simulink model "PubIfDecisionTOS_MDL"  (R2020b)
settings: configuration reference "DspaceConfig" (kept outside this file)
PostLoadFcn:
  | if any(exist('dsrtsu_mdlpostloadfcn', 'file') ~= 0), dsrtsu_mdlpostloadfcn('Execute', bdroot); end
InitFcn:
  | , if any(exist('dsmpb_private', 'file') ~= 0), dsmpb_private('dsmpb_mdlclblib', 'Init', bdroot); end,
undefined symbols (not defined in the file or in its folder): C_TOS_ACCEgoRAxletoFbumplength_m, C_TOS_ACCTargetFront_Flag, C_TOS_AEBJAPedObjDxThre_Val, C_TOS_AEBJAPedObjDyThre_Val, C_TOS_AEBJATargetSize_Val, C_TOS_AEBJAVehObjDxThre_Val, C_TOS_AEBJAVehObjDyThre_Val, C_TOS_AEBJuncPedTargetSize_Val, C_TOS_AEBLatObjDxThre_Val, C_TOS_AEBLatPedDyThre_Val, C_TOS_AEBLatTargetSize_Val, C_TOS_AEBLongTargetInEgoFront_Flag, C_TOS_axAbsGround_Parameter, C_TOS_CameraConfirmedFlag, C_TOS_CNsubjWidth, C_TOS_CurrentLaneCoreMinWidth_Val, C_TOS_CutInProb_Val_Zero, C_TOS_CutOutProb_Val_Zero, C_TOS_D2R_Val, C_TOS_DefaultValueObjectToCenterLine_dy, C_TOS_EgoCarWidth_Val, C_TOS_EgoDxRefPoint_m, C_TOS_EgoRAxletoFbumplength_m, C_TOS_HalfWidthVehicle_Con, C_TOS_HWA_CurrentLaneFlag, C_TOS_HWA_LeftLaneFlag, C_TOS_HWA_MovingDir_Vaild, C_TOS_HWA_MovState_Vaild, C_TOS_HWA_RightLaneFlag, C_TOS_LaneLineCourseErrorFront, C_TOS_LaneLineCourseErrorRear, C_TOS_MotorbikeDefaultWidth_m, C_TOS_NumberOfEffectiveTargets, C_TOS_Obj_Age_Val, C_TOS_Objdx_Constraint_Val, C_TOS_ObjectDefaultWidth_m, C_TOS_ObjInCurrentLane_Val, C_TOS_ObjInCurrentLaneValid, C_TOS_ObjInLeftLaneValid, C_TOS_ObjInRightLaneValid, C_TOS_ObjNotInCurrentLane_Val, C_TOS_ObjNotREElementType, C_TOS_ObjPredictDis_dy_ConstantVal_Zeros, C_TOS_ObjToCenterLine_ConstantVal_Zeros, C_TOS_OFMObjIDInvilad_Val, C_TOS_PIL_LatDisCons_Val_zero, C_TOS_PIL_ObjectCutInFlag_b, C_TOS_PIL_ObjectCutOutFlag_b, C_TOS_PIL_ObjLaneProb_al_Val, C_TOS_PP_ObjFusType_FC_Confirm_b, C_TOS_PP_ObjFusType_FC_FR_Confirm_b, C_TOS_PP_ObjFusType_FR_Confirm_b, C_TOS_RE_80BoolDefault_Val, C_TOS_RE_80Single181Default_Val, C_TOS_RE_80Single255Default_Val, C_TOS_RE_80Uint8Default_Val, C_TOS_RE_D2R, C_TOS_RE_D_180_Val, C_TOS_RE_InvalidObjectID_Val, C_TOS_RE_InvalidTargetChainDir_Val ... (+142)
libraries: simulink x1650, TOS_LIB x361, canfdmsglib x14
(part 49 of 69)

== system PubIfDecisionTOS_MDL/TOS_20201112/TOS_2012080320/TOS/LC_LCKie_ELK/TOS_HWA/CurrentLane/HWA_Object_PreConfirm/TOS_HWA_CurrentLaneFront_TargPreConfirm/TOS_HWA_CurrentLaneFront_TargPreConfirm/Subsystem3 ==
  FR_Confirm : Inport
  Obj_MovingState : Inport  Port=2
  Object_ObstacleProb : Inport  Port=3
  Object_DY : Inport  Port=4
  Chart : Stateflow chart  TreatAsAtomicUnit=on
  Data Type Conversion1 : DataTypeConversion  OutDataTypeStr=Enum: OFM_OBJ_MOVINGSTATE_E
  TOS_HWA_TargetPre_FenceFlag : Outport
  wires:
  Chart/1(ObjectisFence_Flag) -> TOS_HWA_TargetPre_FenceFlag/1
  Object_DY/1 -> Chart/4(Object_DY)
  FR_Confirm/1 -> Chart/1(FR_Confirm)
  Obj_MovingState/1 -> Data Type Conversion1/1
  Object_ObstacleProb/1 -> Chart/3(Object_ObstacleProb)
  Data Type Conversion1/1 -> Chart/2(Obj_MovingState)

== system PubIfDecisionTOS_MDL/TOS_20201112/TOS_2012080320/TOS/LC_LCKie_ELK/TOS_HWA/CurrentLane/HWA_Object_PreConfirm/TOS_HWA_CurrentLaneFront_TargPreConfirm/TOS_HWA_CurrentLaneFront_TargPreConfirm/TOS_HWA_DyConfirm ==
  TOS_HWA_Dy : Inport
  Abs : Abs
  Abs1 : Abs
  Bus Selector3 : BusSelector  OutputSignals=PIL_OverlapRatio,Object_DY,Obj_Dx,Object_ObjType
  Compare To Constant1 : simulink/Logic and Bit Operations/Compare To Constant  relop===  const=OFM_OBJ_TYPE_E.UNKNOWN_TYPE  OutDataTypeStr=boolean
      settings: AttributesFormatString=OFM_OBJ_TYPE_E.UNKNOWN_TYPE = 1
  Compare To Constant2 : simulink/Logic and Bit Operations/Compare To Constant  relop===  const=OFM_OBJ_TYPE_E.MOTORBIKE  OutDataTypeStr=boolean
      settings: AttributesFormatString=OFM_OBJ_TYPE_E.MOTORBIKE = 4
  Compare To Constant3 : simulink/Logic and Bit Operations/Compare To Constant  relop===  const=OFM_OBJ_TYPE_E.PEDESTRIAN  OutDataTypeStr=boolean
      settings: AttributesFormatString=OFM_OBJ_TYPE_E.PEDESTRIAN = 6
  Compare To Constant4 : simulink/Logic and Bit Operations/Compare To Constant  relop===  const=OFM_OBJ_TYPE_E.BICYCLE  OutDataTypeStr=boolean
      settings: AttributesFormatString=OFM_OBJ_TYPE_E.BICYCLE = 5
  Compare To Constant5 : simulink/Logic and Bit Operations/Compare To Constant  relop===  const=OFM_OBJ_TYPE_E.GENERAL_OBJECT  OutDataTypeStr=boolean
      settings: AttributesFormatString=OFM_OBJ_TYPE_E.GENERAL_OBJECT = 7
  Compare To Constant6 : simulink/Logic and Bit Operations/Compare To Constant  relop===  const=OFM_OBJ_TYPE_E.ANIMAL  OutDataTypeStr=boolean
      settings: AttributesFormatString=OFM_OBJ_TYPE_E.ANIMAL = 8
  Compare To Constant7 : simulink/Logic and Bit Operations/Compare To Constant  relop=>=  const=P_TOS_HWA_TargetPre_OverlapThre_Val  OutDataTypeStr=boolean
      settings: AttributesFormatString=P_TOS_HWA_TargetPre_OverlapThre_Val = 0.05
  Data Type Conversion2 : DataTypeConversion  OutDataTypeStr=Enum: OFM_OBJ_TYPE_E
  Logical Operator1 : Logic  Operator=OR  Inputs=6  AllPortsSameDT=off  OutDataTypeStr=boolean
  Logical Operator2 : Logic  Operator=NOT  Inputs=1  AllPortsSameDT=off  OutDataTypeStr=boolean
  Logical Operator3 : Logic  Inputs=3  AllPortsSameDT=off  OutDataTypeStr=boolean
  Logical Operator4 : Logic  AllPortsSameDT=off  OutDataTypeStr=boolean
  Logical Operator6 : Logic  Operator=OR  AllPortsSameDT=off  OutDataTypeStr=boolean
  Relational Operator : RelationalOperator  Operator=<=  OutDataTypeStr=boolean  RndMeth=Simplest
  data3 : Lookup_n-D  NumberOfTableDimensions=1  BreakpointsForDimension1=[0,20,40,60,80,100,120,140]  Table=[1.4,1.4,1.3,1.3,1.2,1.2,1.2,1.2]  RndMeth=Simplest  InputSameDT=on
  TOS_HWA_DyConfirm : Outport
  wires:
  Logical Operator6/1 -> TOS_HWA_DyConfirm/1
  TOS_HWA_Dy/1 -> Bus Selector3/1
  Relational Operator/1 -> Logical Operator3/2
  Abs/1 -> data3/1
  data3/1 -> Relational Operator/2
  Abs1/1 -> Relational Operator/1
  Compare To Constant3/1 -> Logical Operator1/1
  Bus Selector3/2 -> Abs1/1  "<Object_DY>"
  Data Type Conversion2/1 -> Compare To Constant1/1, Compare To Constant2/1, Compare To Constant4/1, Compare To Constant5/1, Compare To Constant6/1, Compare To Constant3/1
  Compare To Constant1/1 -> Logical Operator1/2
  Compare To Constant2/1 -> Logical Operator1/3
  Compare To Constant4/1 -> Logical Operator1/4
  Compare To Constant5/1 -> Logical Operator1/5
  Compare To Constant6/1 -> Logical Operator1/6
  Logical Operator1/1 -> Logical Operator2/1, Logical Operator3/3
  Bus Selector3/3 -> Abs/1  "<Obj_Dx>"
  Bus Selector3/4 -> Data Type Conversion2/1  "<Object_ObjType>"
  Bus Selector3/1 -> Compare To Constant7/1  "<PIL_OverlapRatio>"
  Compare To Constant7/1 -> Logical Operator3/1, Logical Operator4/2
  Logical Operator2/1 -> Logical Operator4/1
  Logical Operator4/1 -> Logical Operator6/1
  Logical Operator3/1 -> Logical Operator6/2

== system PubIfDecisionTOS_MDL/TOS_20201112/TOS_2012080320/TOS/LC_LCKie_ELK/TOS_HWA/LeftLane/HWA_Object_PreConfirm/HWA_Object_PreConfirm/HWA_Object_PreConfirm/  ==
  Object_Type : Inport
  Compare To Constant : simulink/Logic and Bit Operations/Compare To Constant  relop===  const=OFM_OBJ_TYPE_E.CAR  OutDataTypeStr=boolean
      settings: AttributesFormatString=OFM_OBJ_TYPE_E.CAR = 2
  Compare To Constant1 : simulink/Logic and Bit Operations/Compare To Constant  relop===  const=OFM_OBJ_TYPE_E.TRUCK  OutDataTypeStr=boolean
      settings: AttributesFormatString=OFM_OBJ_TYPE_E.TRUCK = 3
  Compare To Constant2 : simulink/Logic and Bit Operations/Compare To Constant  relop===  const=OFM_OBJ_TYPE_E.UNKNOWN_TYPE  OutDataTypeStr=boolean
      settings: AttributesFormatString=OFM_OBJ_TYPE_E.UNKNOWN_TYPE = 1
  Compare To Constant3 : simulink/Logic and Bit Operations/Compare To Constant  relop===  const=OFM_OBJ_TYPE_E.PEDESTRIAN  OutDataTypeStr=boolean
      settings: AttributesFormatString=OFM_OBJ_TYPE_E.PEDESTRIAN = 6
  Compare To Constant4 : simulink/Logic and Bit Operations/Compare To Constant  relop===  const=OFM_OBJ_TYPE_E.MOTORBIKE  OutDataTypeStr=boolean
      settings: AttributesFormatString=OFM_OBJ_TYPE_E.MOTORBIKE = 4
  Compare To Constant5 : simulink/Logic and Bit Operations/Compare To Constant  relop===  const=OFM_OBJ_TYPE_E.BICYCLE  OutDataTypeStr=boolean
      settings: AttributesFormatString=OFM_OBJ_TYPE_E.BICYCLE = 5
  Compare To Constant6 : simulink/Logic and Bit Operations/Compare To Constant  relop===  const=OFM_OBJ_TYPE_E.GENERAL_OBJECT  OutDataTypeStr=boolean
      settings: AttributesFormatString=OFM_OBJ_TYPE_E.GENERAL_OBJECT = 7
  Compare To Constant7 : simulink/Logic and Bit Operations/Compare To Constant  relop===  const=OFM_OBJ_TYPE_E.ANIMAL  OutDataTypeStr=boolean
      settings: AttributesFormatString=OFM_OBJ_TYPE_E.ANIMAL = 8
  Data Type Conversion : DataTypeConversion  OutDataTypeStr=Enum: OFM_OBJ_TYPE_E
  Logical Operator1 : Logic  Operator=OR  Inputs=8  AllPortsSameDT=off  OutDataTypeStr=boolean
  TOS_HWA_TargetPre_ObjType : Outport
  wires:
  Object_Type/1 -> Data Type Conversion/1
  Data Type Conversion/1 -> Compare To Constant6/1, Compare To Constant7/1, Compare To Constant3/1, Compare To Constant5/1, Compare To Constant4/1, Compare To Constant1/1, Compare To Constant/1, Compare To Constant2/1
  Compare To Constant/1 -> Logical Operator1/2
  Compare To Constant1/1 -> Logical Operator1/3
  Compare To Constant4/1 -> Logical Operator1/4
  Compare To Constant5/1 -> Logical Operator1/5
  Logical Operator1/1 -> TOS_HWA_TargetPre_ObjType/1
  Compare To Constant2/1 -> Logical Operator1/1
  Compare To Constant3/1 -> Logical Operator1/6
  Compare To Constant6/1 -> Logical Operator1/7
  Compare To Constant7/1 -> Logical Operator1/8

== system PubIfDecisionTOS_MDL/TOS_20201112/TOS_2012080320/TOS/LC_LCKie_ELK/TOS_HWA/LeftLane/HWA_Object_PreConfirm/HWA_Object_PreConfirm/HWA_Object_PreConfirm/Subsystem ==
  PP_ObjFusType_FC_FR_Confirm : Inport
  PP_ObjFusType_FR_Confirm : Inport  Port=2
  PP_ObjFusType_FC_Confirm : Inport  Port=3
  Compare To Constant1 : simulink/Logic and Bit Operations/Compare To Constant  relop===  const=C_TOS_PP_ObjFusType_FC_Confirm_b  OutDataTypeStr=boolean
      settings: AttributesFormatString=C_TOS_PP_ObjFusType_FC_Confirm_b = 1
  Compare To Constant5 : simulink/Logic and Bit Operations/Compare To Constant  relop===  const=C_TOS_PP_ObjFusType_FC_FR_Confirm_b  OutDataTypeStr=boolean
      settings: AttributesFormatString=C_TOS_PP_ObjFusType_FC_FR_Confirm_b = 1
  Compare To Constant6 : simulink/Logic and Bit Operations/Compare To Constant  relop===  const=C_TOS_PP_ObjFusType_FR_Confirm_b  OutDataTypeStr=boolean
      settings: AttributesFormatString=C_TOS_PP_ObjFusType_FR_Confirm_b = 1
  Logical Operator : Logic  Operator=OR  Inputs=3  AllPortsSameDT=off  OutDataTypeStr=boolean
  TOS_HWA_TargetPre_TargetFusionTypeFlag : Outport
  wires:
  Logical Operator/1 -> TOS_HWA_TargetPre_TargetFusionTypeFlag/1
  Compare To Constant1/1 -> Logical Operator/3
  Compare To Constant6/1 -> Logical Operator/2
  PP_ObjFusType_FC_FR_Confirm/1 -> Compare To Constant5/1
  PP_ObjFusType_FC_Confirm/1 -> Compare To Constant1/1
  PP_ObjFusType_FR_Confirm/1 -> Compare To Constant6/1
  Compare To Constant5/1 -> Logical Operator/1

== system PubIfDecisionTOS_MDL/TOS_20201112/TOS_2012080320/TOS/LC_LCKie_ELK/TOS_HWA/LeftLane/HWA_Object_PreConfirm/HWA_Object_PreConfirm/HWA_Object_PreConfirm/Subsystem1 ==
  note: 静止目标 、必须有摄像头参与
  PP_ObjFusType_FC_Confirm : Inport
  Obj_MovingState : Inport  Port=2
  Compare To Constant2 : simulink/Logic and Bit Operations/Compare To Constant  relop===  const=OFM_OBJ_MOVINGSTATE_E.UNKNOWN  OutDataTypeStr=boolean
      settings: AttributesFormatString=OFM_OBJ_MOVINGSTATE_E.UNKNOWN = 1
  Compare To Constant3 : simulink/Logic and Bit Operations/Compare To Constant  relop===  const=OFM_OBJ_MOVINGSTATE_E.STATIONARY  OutDataTypeStr=boolean
      settings: AttributesFormatString=OFM_OBJ_MOVINGSTATE_E.STATIONARY = 3
  Compare To Constant5 : simulink/Logic and Bit Operations/Compare To Constant  relop===  const=C_TOS_PP_ObjFusType_FC_Confirm_b  OutDataTypeStr=boolean
      settings: AttributesFormatString=C_TOS_PP_ObjFusType_FC_Confirm_b = 1
  Constant : Constant  OutDataTypeStr=boolean
  Data Type Conversion1 : DataTypeConversion  OutDataTypeStr=Enum: OFM_OBJ_MOVINGSTATE_E
  Logical Operator : Logic  AllPortsSameDT=off  OutDataTypeStr=boolean
  Logical Operator4 : Logic  Operator=OR  AllPortsSameDT=off  OutDataTypeStr=boolean
  Switch : Switch  Criteria=u2 > Threshold
  TOS_HWA_TargetPre_ObjectPassedbyTarget_Flag : Outport
  wires:
  Switch/1 -> TOS_HWA_TargetPre_ObjectPassedbyTarget_Flag/1
  Compare To Constant3/1 -> Logical Operator4/1
  Obj_MovingState/1 -> Data Type Conversion1/1
  Data Type Conversion1/1 -> Compare To Constant2/1, Compare To Constant3/1
  PP_ObjFusType_FC_Confirm/1 -> Compare To Constant5/1
  Compare To Constant5/1 -> Logical Operator/1
  Compare To Constant2/1 -> Logical Operator4/2
  Logical Operator4/1 -> Logical Operator/2, Switch/2
  Logical Operator/1 -> Switch/1
  Constant/1 -> Switch/3

== system PubIfDecisionTOS_MDL/TOS_20201112/TOS_2012080320/TOS/LC_LCKie_ELK/TOS_HWA/LeftLane/HWA_Object_PreConfirm/HWA_Object_PreConfirm/HWA_Object_PreConfirm/TOS_HWA_DyConfirm ==
  TOS_HWA_Dy : Inport
  Abs : Abs
  Abs1 : Abs
  Bus Selector3 : BusSelector  OutputSignals=Object_DY,Obj_Dx,Object_ObjType
  Compare To Constant : simulink/Logic and Bit Operations/Compare To Constant  relop===  const=OFM_OBJ_TYPE_E.CAR  OutDataTypeStr=boolean
      settings: AttributesFormatString=OFM_OBJ_TYPE_E.CAR = 2
  Compare To Constant1 : simulink/Logic and Bit Operations/Compare To Constant  relop===  const=OFM_OBJ_TYPE_E.TRUCK  OutDataTypeStr=boolean
      settings: AttributesFormatString=OFM_OBJ_TYPE_E.TRUCK = 3
  Compare To Constant4 : simulink/Logic and Bit Operations/Compare To Constant  relop===  const=OFM_OBJ_TYPE_E.MOTORBIKE  OutDataTypeStr=boolean
      settings: AttributesFormatString=OFM_OBJ_TYPE_E.MOTORBIKE = 4
  Compare To Constant5 : simulink/Logic and Bit Operations/Compare To Constant  relop===  const=OFM_OBJ_TYPE_E.BICYCLE  OutDataTypeStr=boolean
      settings: AttributesFormatString=OFM_OBJ_TYPE_E.BICYCLE = 5
  Data Type Conversion2 : DataTypeConversion  OutDataTypeStr=Enum: OFM_OBJ_TYPE_E
  Logical Operator1 : Logic  Operator=OR  Inputs=4  AllPortsSameDT=off  OutDataTypeStr=boolean
  Logical Operator2 : Logic  Operator=OR  AllPortsSameDT=off  OutDataTypeStr=boolean
  Relational Operator : RelationalOperator  Operator=<=  OutDataTypeStr=boolean  RndMeth=Simplest
  data3 : Lookup_n-D  NumberOfTableDimensions=1  BreakpointsForDimension1=[0,20,40,60,80,100,120,140]  Table=[1.4,1.4,1.3,1.3,1.2,1.2,1.2,1.2]  RndMeth=Simplest  InputSameDT=on
  TOS_HWA_TargetPre_DyConfirm : Outport
  wires:
  Logical Operator2/1 -> TOS_HWA_TargetPre_DyConfirm/1
  TOS_HWA_Dy/1 -> Bus Selector3/1
  Relational Operator/1 -> Logical Operator2/1
  Abs/1 -> data3/1
  data3/1 -> Relational Operator/2
  Abs1/1 -> Relational Operator/1
  Bus Selector3/1 -> Abs1/1  "<Object_DY>"
  Data Type Conversion2/1 -> Compare To Constant/1, Compare To Constant5/1, Compare To Constant4/1, Compare To Constant1/1
  Logical Operator1/1 -> Logical Operator2/2
  Bus Selector3/2 -> Abs/1  "<Obj_Dx>"
  Bus Selector3/3 -> Data Type Conversion2/1  "<Object_ObjType>"
  Compare To Constant/1 -> Logical Operator1/1
  Compare To Constant1/1 -> Logical Operator1/2
  Compare To Constant4/1 -> Logical Operator1/3
  Compare To Constant5/1 -> Logical Operator1/4

== system PubIfDecisionTOS_MDL/TOS_20201112/TOS_2012080320/TOS/LC_LCKie_ELK/TOS_HWA/LeftLane/TOS_HWA_LeftLane/TOS_HWA_LeftLane/TOS_HWA/HWA_LeftLane ==
  Object_VX : Inport
  Object_VY : Inport  Port=2
  object_MovingState : Inport  Port=3
  PP_ObjMovingDirSignalProcessing : Inport  Port=4
  Object_HeadingAngle : Inport  Port=5
  Object_Type : Inport  Port=6
  TOS_TLJ_LeftLaneConfirm_Flag : Inport  Port=7
  Object_DX : Inport  Port=8
  Object_DY : Inport  Port=9
  Object_Fus_Type : Inport  Port=10
  PP_ObjFusType_FC_FR_Confirm : Inport  Port=11
  PP_ObjFusType_FR_Confirm : Inport  Port=12
  PP_ObjFusType_FC_Confirm : Inport  Port=13
  VIE_EgoVelocity : Inport  Port=14
  Bus Creator : BusCreator  Inputs=14
  Bus Creator1 : BusCreator  Inputs=3
  Bus Creator2 : BusCreator  Inputs=10
  Bus Creator3 : BusCreator  Inputs=10
  Bus Creator4 : BusCreator  Inputs=10
  Bus Selector : BusSelector  OutputSignals=object_MovingState,PP_ObjMovingDirSignalProcessing,Object_HeadingAngle,Object_VX,Object_VY,VIE_EgoVelocity
  Bus Selector1 : BusSelector  OutputSignals=Object_VX,Object_VY,VIE_EgoVelocity
  Bus Selector2 : BusSelector  OutputSignals=HWA_MovState_InternalSig,HWA_InternalSig.Object_Fus_Type,HWA_InternalSig.TOS_TLJ_LeftLaneConfirm_Flag,HWA_MovingDir_InternalSig,HWA_InternalSig.Object_DY,HWA_InternalSig.Object_DX
  Bus Selector3 : BusSelector  OutputSignals=HWA_InternalSig.object_MovingState,HWA_InternalSig.PP_ObjFusType_FR_Confirm,HWA_InternalSig.PP_ObjFusType_FC_Confirm,HWA_MovState_InternalSig,HWA_InternalSig.TOS_TLJ_LeftLaneConfirm_Flag,HWA_MovingDir_InternalSig,HWA_InternalSig.Object_DX
  Bus Selector4 : BusSelector  OutputSignals=HWA_InternalSig.Object_DX
  Bus Selector5 : BusSelector  OutputSignals=HWA_InternalSig.Object_DX
  Bus Selector6 : BusSelector  OutputSignals=TOS_HWA_LeftFront_TargConfirm_b,TOS_HWA_LeftRear_TargConfirm_b,TOS_HWA_LeftFront_FusType_ObserVale,TOS_HWA_InLeftLane_Front_Flag_ObserVale,TOS_HWA_LeftFront_TargMovDir_ObserVale,TOS_HWA_LeftRear_MovState_ObserVale,TOS_HWA_LeftRear_FusionType_ObserVale,TOS_HWA_InLeftLane_Rear_Flag_ObserVale,TOS_HWA_LeftRear_TargetMovingDir_ObserVale,TOS_HWA_LeftRear_DyConfirm_ObserVale
  Compare To Constant1 : simulink/Logic and Bit Operations/Compare To Constant  relop=<=  const=P_TOS_EgoFrontDxThre_Val  OutDataTypeStr=boolean
      settings: AttributesFormatString=P_TOS_EgoFrontDxThre_Val = 120
  Compare To Constant14 : simulink/Logic and Bit Operations/Compare To Constant  relop=<  const=P_TOS_RefPoint_dx_m  OutDataTypeStr=boolean
      settings: AttributesFormatString=P_TOS_RefPoint_dx_m = 0
  Compare To Constant2 : simulink/Logic and Bit Operations/Compare To Constant  relop=>=  const=P_TOS_RefPoint_dx_m  OutDataTypeStr=boolean
      settings: AttributesFormatString=P_TOS_RefPoint_dx_m = 0
  Compare To Constant3 : simulink/Logic and Bit Operations/Compare To Constant  relop=>=  const=P_TOS_EgoRearDxThre_Val  OutDataTypeStr=boolean
      settings: AttributesFormatString=P_TOS_EgoRearDxThre_Val = -80
  HWA_LeftLane_Default : Subsystem
  HWA_LeftLane_Front : Subsystem
  HWA_LeftLane_Rear : Subsystem
  HWA_MovState : Subsystem
  HWA_MovingDir : Subsystem
  Logical Operator1 : Logic  AllPortsSameDT=off  OutDataTypeStr=boolean
  Logical Operator2 : Logic  AllPortsSameDT=off  OutDataTypeStr=boolean
  Logical Operator3 : Logic  Operator=OR  AllPortsSameDT=off  OutDataTypeStr=boolean
  Switch : Switch  Criteria=u2 > Threshold
  Switch1 : Switch  Criteria=u2 > Threshold
  TOS_HWA_TargetInLeftLane_b : Outport
  TOS_HWA_LeftFront_TargConfirm_b : Outport  Port=2
  TOS_HWA_LeftRear_TargConfirm_b : Outport  Port=3
  TOS_HWA_LeftFront_FusType_ObserVale : Outport  Port=4
  TOS_HWA_InLeftLane_Front_Flag_ObserVale : Outport  Port=5
  TOS_HWA_LeftFront_TargMovDir_ObserVale : Outport  Port=6
  TOS_HWA_LeftRear_MovState_ObserVale : Outport  Port=7
  TOS_HWA_LeftRear_FusionType_ObserVale : Outport  Port=8
  TOS_HWA_InLeftLane_Rear_Flag_ObserVale : Outport  Port=9
  TOS_HWA_LeftRear_TargetMovingDir_ObserVale : Outport  Port=10
  TOS_HWA_LeftRear_DyConfirm_ObserVale : Outport  Port=11
  wires:
  Bus Selector3/7 -> HWA_LeftLane_Front/7(Object_DX)  "<Object_DX>"
  Logical Operator3/1 -> TOS_HWA_TargetInLeftLane_b/1
  Bus Selector6/10 -> TOS_HWA_LeftRear_DyConfirm_ObserVale/1  "<TOS_HWA_LeftRear_DyConfirm_ObserVale>"
  Bus Selector6/9 -> TOS_HWA_LeftRear_TargetMovingDir_ObserVale/1  "<TOS_HWA_LeftRear_TargetMovingDir_ObserVale>"
  Bus Selector6/8 -> TOS_HWA_InLeftLane_Rear_Flag_ObserVale/1  "<TOS_HWA_InLeftLane_Rear_Flag_ObserVale>"
  Bus Selector6/7 -> TOS_HWA_LeftRear_FusionType_ObserVale/1  "<TOS_HWA_LeftRear_FusionType_ObserVale>"
  Bus Selector6/6 -> TOS_HWA_LeftRear_MovState_ObserVale/1  "<TOS_HWA_LeftRear_MovState_ObserVale>"
  Bus Selector6/5 -> TOS_HWA_LeftFront_TargMovDir_ObserVale/1  "<TOS_HWA_LeftFront_TargMovDir_ObserVale>"
  Bus Selector6/4 -> TOS_HWA_InLeftLane_Front_Flag_ObserVale/1  "<TOS_HWA_InLeftLane_Front_Flag_ObserVale>"
  Bus Selector6/3 -> TOS_HWA_LeftFront_FusType_ObserVale/1  "<TOS_HWA_LeftFront_FusType_ObserVale>"
  Bus Selector6/2 -> TOS_HWA_LeftRear_TargConfirm_b/1, Logical Operator3/2  "<TOS_HWA_LeftRear_TargConfirm_b>"
  Bus Selector6/1 -> TOS_HWA_LeftFront_TargConfirm_b/1, Logical Operator3/1  "<TOS_HWA_LeftFront_TargConfirm_b>"
  Switch/1 -> Bus Selector6/1
  Bus Creator4/1 -> Switch1/3
  Switch1/1 -> Switch/3
  Bus Creator3/1 -> Switch1/1
  Bus Creator2/1 -> Switch/1
  Bus Selector4/1 -> Compare To Constant3/1, Compare To Constant14/1  "<Object_DX>"
  Bus Selector2/6 -> HWA_LeftLane_Rear/6(Object_DX)  "<Object_DX>"
  Bus Selector3/6 -> HWA_LeftLane_Front/6(HWA_MovingDir_InternalSig)  "<HWA_MovingDir_InternalSig>"
  Bus Selector3/5 -> HWA_LeftLane_Front/5(TOS_TLJ_LeftLaneConfirm_Flag)  "<TOS_TLJ_LeftLaneConfirm_Flag>"
  Bus Selector3/4 -> HWA_LeftLane_Front/4(HWA_MovState_InternalSig)  "<HWA_MovState_InternalSig>"
  Bus Selector3/3 -> HWA_LeftLane_Front/3(PP_ObjFusType_FC_Confirm)  "<PP_ObjFusType_FC_Confirm>"
  Bus Selector3/2 -> HWA_LeftLane_Front/2(PP_ObjFusType_FR_Confirm)  "<PP_ObjFusType_FR_Confirm>"
  Bus Selector3/1 -> HWA_LeftLane_Front/1(object_MovingState)  "<object_MovingState>"
  Bus Selector2/1 -> HWA_LeftLane_Rear/1(HWA_MovState_InternalSig)  "<HWA_MovState_InternalSig>"
  Bus Selector2/2 -> HWA_LeftLane_Rear/2(Object_Fus_Type)  "<Object_Fus_Type>"
  Bus Selector2/3 -> HWA_LeftLane_Rear/3(TOS_TLJ_LeftLaneConfirm_Flag)  "<TOS_TLJ_LeftLaneConfirm_Flag>"
  Bus Selector2/4 -> HWA_LeftLane_Rear/4(HWA_MovingDir_InternalSig)  "<HWA_MovingDir_InternalSig>"
  Bus Selector2/5 -> HWA_LeftLane_Rear/5(Object_DY)  "<Object_DY>"
  Object_DY/1 -> Bus Creator/9  "Object_DY"
  Bus Creator1/1 -> Bus Selector3/1, Bus Selector5/1, Bus Selector2/1, Bus Selector4/1
  HWA_MovingDir/1(HWA_MovingDir_InternalSig) -> Bus Creator1/2  "HWA_MovingDir_InternalSig"
  HWA_MovState/1(HWA_MovState_InternalSig) -> Bus Creator1/3  "HWA_MovState_InternalSig"
  Bus Selector1/3 -> HWA_MovState/3(VIE_EgoVelocity)  "<VIE_EgoVelocity>"
  Bus Selector1/2 -> HWA_MovState/2(Object_VY)  "<Object_VY>"
  Bus Selector1/1 -> HWA_MovState/1(Object_VX)  "<Object_VX>"
  Bus Selector/6 -> HWA_MovingDir/6(VIE_EgoVelocity)  "<VIE_EgoVelocity>"
  Bus Selector/5 -> HWA_MovingDir/5(Object_VY)  "<Object_VY>"
  Bus Selector/4 -> HWA_MovingDir/4(Object_VX)  "<Object_VX>"
  Bus Selector/3 -> HWA_MovingDir/3(Object_HeadingAngle)  "<Object_HeadingAngle>"
  Bus Selector/2 -> HWA_MovingDir/2(PP_ObjMovingDirSignalProcessing)  "<PP_ObjMovingDirSignalProcessing>"
  Bus Selector/1 -> HWA_MovingDir/1(object_MovingState)  "<object_MovingState>"
  Bus Creator/1 -> Bus Creator1/1, Bus Selector/1, Bus Selector1/1  "HWA_InternalSig"
  PP_ObjFusType_FR_Confirm/1 -> Bus Creator/12  "PP_ObjFusType_FR_Confirm"
  PP_ObjFusType_FC_FR_Confirm/1 -> Bus Creator/11  "PP_ObjFusType_FC_FR_Confirm"
  Object_Fus_Type/1 -> Bus Creator/10  "Object_Fus_Type"
  Object_DX/1 -> Bus Creator/8  "Object_DX"
  TOS_TLJ_LeftLaneConfirm_Flag/1 -> Bus Creator/7  "TOS_TLJ_LeftLaneConfirm_Flag"
  Object_Type/1 -> Bus Creator/6  "Object_Type"
  Object_HeadingAngle/1 -> Bus Creator/5  "Object_HeadingAngle"
  PP_ObjMovingDirSignalProcessing/1 -> Bus Creator/4  "PP_ObjMovingDirSignalProcessing"
  object_MovingState/1 -> Bus Creator/3  "object_MovingState"
  Object_VY/1 -> Bus Creator/2  "Object_VY"
  VIE_EgoVelocity/1 -> Bus Creator/14  "VIE_EgoVelocity"
  Object_VX/1 -> Bus Creator/1  "Object_VX"
  Logical Operator2/1 -> Switch/2
  Logical Operator1/1 -> Switch1/2
  Compare To Constant1/1 -> Logical Operator2/2
  Compare To Constant2/1 -> Logical Operator2/1
  Compare To Constant14/1 -> Logical Operator1/2
  Compare To Constant3/1 -> Logical Operator1/1
  Bus Selector5/1 -> Compare To Constant2/1, Compare To Constant1/1  "<Object_DX>"
  PP_ObjFusType_FC_Confirm/1 -> Bus Creator/13  "PP_ObjFusType_FC_Confirm"
  HWA_LeftLane_Front/1(TOS_HWA_LeftFront_TargConfirm_b) -> Bus Creator2/1
  HWA_LeftLane_Front/2(TOS_HWA_LeftFront_FusType_ObserVale) -> Bus Creator2/2
  HWA_LeftLane_Front/3(TOS_HWA_InLeftLane_Front_Flag_ObserVale) -> Bus Creator2/3
  HWA_LeftLane_Front/4(TOS_HWA_LeftFront_TargMovDir_ObserVale) -> Bus Creator2/4
  HWA_LeftLane_Front/5(TOS_HWA_LeftRear_TargConfirm_b) -> Bus Creator2/5
  HWA_LeftLane_Front/6(TOS_HWA_LeftRear_MovState_ObserVale) -> Bus Creator2/6
  HWA_LeftLane_Front/7(TOS_HWA_LeftRear_FusionType_ObserVale) -> Bus Creator2/7
  HWA_LeftLane_Front/8(TOS_HWA_InLeftLane_Rear_Flag_ObserVale) -> Bus Creator2/8
  HWA_LeftLane_Front/9(TOS_HWA_LeftRear_TargetMovingDir_ObserVale) -> Bus Creator2/9
  HWA_LeftLane_Front/10(TOS_HWA_LeftRear_DyConfirm_ObserVale) -> Bus Creator2/10
  HWA_LeftLane_Rear/1(TOS_HWA_LeftFront_TargConfirm_b) -> Bus Creator3/1
  HWA_LeftLane_Rear/2(TOS_HWA_LeftFront_FusType_ObserVale) -> Bus Creator3/2
  HWA_LeftLane_Rear/3(TOS_HWA_InLeftLane_Front_Flag_ObserVale) -> Bus Creator3/3
  HWA_LeftLane_Rear/4(TOS_HWA_LeftFront_TargMovDir_ObserVale) -> Bus Creator3/4
  HWA_LeftLane_Rear/5(TOS_HWA_LeftRear_TargConfirm_b) -> Bus Creator3/5
  HWA_LeftLane_Rear/6(TOS_HWA_LeftRear_MovState_ObserVale) -> Bus Creator3/6
  HWA_LeftLane_Rear/7(TOS_HWA_LeftRear_FusionType_ObserVale) -> Bus Creator3/7
  HWA_LeftLane_Rear/8(TOS_HWA_InLeftLane_Rear_Flag_ObserVale) -> Bus Creator3/8
  HWA_LeftLane_Rear/9(TOS_HWA_LeftRear_TargetMovingDir_ObserVale) -> Bus Creator3/9
  HWA_LeftLane_Rear/10(TOS_HWA_LeftRear_DyConfirm_ObserVale) -> Bus Creator3/10
  HWA_LeftLane_Default/3(TOS_HWA_InLeftLane_Front_Flag_ObserVale) -> Bus Creator4/3
  HWA_LeftLane_Default/2(TOS_HWA_LeftFront_FusType_ObserVale) -> Bus Creator4/2
  HWA_LeftLane_Default/4(TOS_HWA_LeftFront_TargMovDir_ObserVale) -> Bus Creator4/4
  HWA_LeftLane_Default/1(TOS_HWA_LeftFront_TargConfirm_b) -> Bus Creator4/1
  HWA_LeftLane_Default/5(TOS_HWA_LeftRear_TargConfirm_b) -> Bus Creator4/5
  HWA_LeftLane_Default/6(TOS_HWA_LeftRear_MovState_ObserVale) -> Bus Creator4/6
  HWA_LeftLane_Default/7(TOS_HWA_LeftRear_FusionType_ObserVale) -> Bus Creator4/7
  HWA_LeftLane_Default/8(TOS_HWA_InLeftLane_Rear_Flag_ObserVale) -> Bus Creator4/8
  HWA_LeftLane_Default/9(TOS_HWA_LeftRear_TargetMovingDir_ObserVale) -> Bus Creator4/9
  HWA_LeftLane_Default/10(TOS_HWA_LeftRear_DyConfirm_ObserVale) -> Bus Creator4/10

== system PubIfDecisionTOS_MDL/TOS_20201112/TOS_2012080320/TOS/LC_LCKie_ELK/TOS_HWA/RightLane/HWA_Object_PreConfirm/HWA_Object_PreConfirm/HWA_Object_PreConfirm/  ==
  Object_Type : Inport
  Compare To Constant : simulink/Logic and Bit Operations/Compare To Constant  relop===  const=OFM_OBJ_TYPE_E.CAR  OutDataTypeStr=boolean
      settings: AttributesFormatString=OFM_OBJ_TYPE_E.CAR = 2
  Compare To Constant1 : simulink/Logic and Bit Operations/Compare To Constant  relop===  const=OFM_OBJ_TYPE_E.TRUCK  OutDataTypeStr=boolean
      settings: AttributesFormatString=OFM_OBJ_TYPE_E.TRUCK = 3
  Compare To Constant2 : simulink/Logic and Bit Operations/Compare To Constant  relop===  const=OFM_OBJ_TYPE_E.UNKNOWN_TYPE  OutDataTypeStr=boolean
      settings: AttributesFormatString=OFM_OBJ_TYPE_E.UNKNOWN_TYPE = 1
  Compare To Constant3 : simulink/Logic and Bit Operations/Compare To Constant  relop===  const=OFM_OBJ_TYPE_E.PEDESTRIAN  OutDataTypeStr=boolean
      settings: AttributesFormatString=OFM_OBJ_TYPE_E.PEDESTRIAN = 6
  Compare To Constant4 : simulink/Logic and Bit Operations/Compare To Constant  relop===  const=OFM_OBJ_TYPE_E.MOTORBIKE  OutDataTypeStr=boolean
      settings: AttributesFormatString=OFM_OBJ_TYPE_E.MOTORBIKE = 4
  Compare To Constant5 : simulink/Logic and Bit Operations/Compare To Constant  relop===  const=OFM_OBJ_TYPE_E.BICYCLE  OutDataTypeStr=boolean
      settings: AttributesFormatString=OFM_OBJ_TYPE_E.BICYCLE = 5
  Compare To Constant6 : simulink/Logic and Bit Operations/Compare To Constant  relop===  const=OFM_OBJ_TYPE_E.GENERAL_OBJECT  OutDataTypeStr=boolean
      settings: AttributesFormatString=OFM_OBJ_TYPE_E.GENERAL_OBJECT = 7
  Compare To Constant7 : simulink/Logic and Bit Operations/Compare To Constant  relop===  const=OFM_OBJ_TYPE_E.ANIMAL  OutDataTypeStr=boolean
      settings: AttributesFormatString=OFM_OBJ_TYPE_E.ANIMAL = 8
  Data Type Conversion : DataTypeConversion  OutDataTypeStr=Enum: OFM_OBJ_TYPE_E
  Logical Operator1 : Logic  Operator=OR  Inputs=8  AllPortsSameDT=off  OutDataTypeStr=boolean
  TOS_HWA_TargetPre_ObjType : Outport
  wires:
  Object_Type/1 -> Data Type Conversion/1
  Data Type Conversion/1 -> Compare To Constant6/1, Compare To Constant7/1, Compare To Constant3/1, Compare To Constant5/1, Compare To Constant4/1, Compare To Constant1/1, Compare To Constant/1, Compare To Constant2/1
  Compare To Constant/1 -> Logical Operator1/2
  Compare To Constant1/1 -> Logical Operator1/3
  Compare To Constant4/1 -> Logical Operator1/4
  Compare To Constant5/1 -> Logical Operator1/5
  Logical Operator1/1 -> TOS_HWA_TargetPre_ObjType/1
  Compare To Constant2/1 -> Logical Operator1/1
  Compare To Constant3/1 -> Logical Operator1/6
  Compare To Constant6/1 -> Logical Operator1/7
  Compare To Constant7/1 -> Logical Operator1/8

== system PubIfDecisionTOS_MDL/TOS_20201112/TOS_2012080320/TOS/LC_LCKie_ELK/TOS_HWA/RightLane/HWA_Object_PreConfirm/HWA_Object_PreConfirm/HWA_Object_PreConfirm/Subsystem ==
  PP_ObjFusType_FC_FR_Confirm : Inport
  PP_ObjFusType_FR_Confirm : Inport  Port=2
  PP_ObjFusType_FC_Confirm : Inport  Port=3
  Compare To Constant1 : simulink/Logic and Bit Operations/Compare To Constant  relop===  const=C_TOS_PP_ObjFusType_FC_Confirm_b  OutDataTypeStr=boolean
      settings: AttributesFormatString=C_TOS_PP_ObjFusType_FC_Confirm_b = 1
  Compare To Constant5 : simulink/Logic and Bit Operations/Compare To Constant  relop===  const=C_TOS_PP_ObjFusType_FC_FR_Confirm_b  OutDataTypeStr=boolean
      settings: AttributesFormatString=C_TOS_PP_ObjFusType_FC_FR_Confirm_b = 1
  Compare To Constant6 : simulink/Logic and Bit Operations/Compare To Constant  relop===  const=C_TOS_PP_ObjFusType_FR_Confirm_b  OutDataTypeStr=boolean
      settings: AttributesFormatString=C_TOS_PP_ObjFusType_FR_Confirm_b = 1
  Logical Operator : Logic  Operator=OR  Inputs=3  AllPortsSameDT=off  OutDataTypeStr=boolean
  TOS_HWA_TargetPre_TargetFusionTypeFlag : Outport
  wires:
  Logical Operator/1 -> TOS_HWA_TargetPre_TargetFusionTypeFlag/1
  Compare To Constant1/1 -> Logical Operator/3
  Compare To Constant6/1 -> Logical Operator/2
  PP_ObjFusType_FC_FR_Confirm/1 -> Compare To Constant5/1
  PP_ObjFusType_FC_Confirm/1 -> Compare To Constant1/1
  PP_ObjFusType_FR_Confirm/1 -> Compare To Constant6/1
  Compare To Constant5/1 -> Logical Operator/1

== system PubIfDecisionTOS_MDL/TOS_20201112/TOS_2012080320/TOS/LC_LCKie_ELK/TOS_HWA/RightLane/HWA_Object_PreConfirm/HWA_Object_PreConfirm/HWA_Object_PreConfirm/Subsystem1 ==
  note: 静止目标 、必须有摄像头参与
  PP_ObjFusType_FC_Confirm : Inport
  Obj_MovingState : Inport  Port=2
  Compare To Constant2 : simulink/Logic and Bit Operations/Compare To Constant  relop===  const=OFM_OBJ_MOVINGSTATE_E.UNKNOWN  OutDataTypeStr=boolean
      settings: AttributesFormatString=OFM_OBJ_MOVINGSTATE_E.UNKNOWN = 1
  Compare To Constant3 : simulink/Logic and Bit Operations/Compare To Constant  relop===  const=OFM_OBJ_MOVINGSTATE_E.STATIONARY  OutDataTypeStr=boolean
      settings: AttributesFormatString=OFM_OBJ_MOVINGSTATE_E.STATIONARY = 3
  Compare To Constant5 : simulink/Logic and Bit Operations/Compare To Constant  relop===  const=C_TOS_PP_ObjFusType_FC_Confirm_b  OutDataTypeStr=boolean
      settings: AttributesFormatString=C_TOS_PP_ObjFusType_FC_Confirm_b = 1
  Constant : Constant  OutDataTypeStr=boolean
  Data Type Conversion1 : DataTypeConversion  OutDataTypeStr=Enum: OFM_OBJ_MOVINGSTATE_E
  Logical Operator : Logic  AllPortsSameDT=off  OutDataTypeStr=boolean
  Logical Operator4 : Logic  Operator=OR  AllPortsSameDT=off  OutDataTypeStr=boolean
  Switch : Switch  Criteria=u2 > Threshold
  TOS_HWA_TargetPre_ObjectPassedbyTarget_Flag : Outport
  wires:
  Switch/1 -> TOS_HWA_TargetPre_ObjectPassedbyTarget_Flag/1
  Compare To Constant3/1 -> Logical Operator4/1
  Obj_MovingState/1 -> Data Type Conversion1/1
  Data Type Conversion1/1 -> Compare To Constant2/1, Compare To Constant3/1
  PP_ObjFusType_FC_Confirm/1 -> Compare To Constant5/1
  Compare To Constant5/1 -> Logical Operator/1
  Compare To Constant2/1 -> Logical Operator4/2
  Logical Operator4/1 -> Logical Operator/2, Switch/2
  Logical Operator/1 -> Switch/1
  Constant/1 -> Switch/3

== system PubIfDecisionTOS_MDL/TOS_20201112/TOS_2012080320/TOS/LC_LCKie_ELK/TOS_HWA/RightLane/HWA_Object_PreConfirm/HWA_Object_PreConfirm/HWA_Object_PreConfirm/TOS_HWA_DyConfirm ==
  TOS_HWA_Dy : Inport
  Abs : Abs
  Abs1 : Abs
  Bus Selector3 : BusSelector  OutputSignals=Object_DY,Obj_Dx,Object_ObjType
  Compare To Constant : simulink/Logic and Bit Operations/Compare To Constant  relop===  const=OFM_OBJ_TYPE_E.CAR  OutDataTypeStr=boolean
      settings: AttributesFormatString=OFM_OBJ_TYPE_E.CAR = 2
  Compare To Constant1 : simulink/Logic and Bit Operations/Compare To Constant  relop===  const=OFM_OBJ_TYPE_E.TRUCK  OutDataTypeStr=boolean
      settings: AttributesFormatString=OFM_OBJ_TYPE_E.TRUCK = 3
  Compare To Constant4 : simulink/Logic and Bit Operations/Compare To Constant  relop===  const=OFM_OBJ_TYPE_E.MOTORBIKE  OutDataTypeStr=boolean
      settings: AttributesFormatString=OFM_OBJ_TYPE_E.MOTORBIKE = 4
  Compare To Constant5 : simulink/Logic and Bit Operations/Compare To Constant  relop===  const=OFM_OBJ_TYPE_E.BICYCLE  OutDataTypeStr=boolean
      settings: AttributesFormatString=OFM_OBJ_TYPE_E.BICYCLE = 5
  Data Type Conversion2 : DataTypeConversion  OutDataTypeStr=Enum: OFM_OBJ_TYPE_E
  Logical Operator1 : Logic  Operator=OR  Inputs=4  AllPortsSameDT=off  OutDataTypeStr=boolean
  Logical Operator2 : Logic  Operator=OR  AllPortsSameDT=off  OutDataTypeStr=boolean
  Relational Operator : RelationalOperator  Operator=<=  OutDataTypeStr=boolean  RndMeth=Simplest
  data3 : Lookup_n-D  NumberOfTableDimensions=1  BreakpointsForDimension1=[0,20,40,60,80,100,120,140]  Table=[1.4,1.4,1.3,1.3,1.2,1.2,1.2,1.2]  RndMeth=Simplest  InputSameDT=on
  TOS_HWA_TargetPre_DyConfirm : Outport
  wires:
  Logical Operator2/1 -> TOS_HWA_TargetPre_DyConfirm/1
  TOS_HWA_Dy/1 -> Bus Selector3/1
  Relational Operator/1 -> Logical Operator2/1
  Abs/1 -> data3/1
  data3/1 -> Relational Operator/2
  Abs1/1 -> Relational Operator/1
  Bus Selector3/1 -> Abs1/1  "<Object_DY>"
  Data Type Conversion2/1 -> Compare To Constant/1, Compare To Constant5/1, Compare To Constant4/1, Compare To Constant1/1
  Logical Operator1/1 -> Logical Operator2/2
  Bus Selector3/2 -> Abs/1  "<Obj_Dx>"
  Bus Selector3/3 -> Data Type Conversion2/1  "<Object_ObjType>"
  Compare To Constant/1 -> Logical Operator1/1
  Compare To Constant1/1 -> Logical Operator1/2
  Compare To Constant4/1 -> Logical Operator1/3
  Compare To Constant5/1 -> Logical Operator1/4

== system PubIfDecisionTOS_MDL/TOS_20201112/TOS_2012080320/TOS/LC_LCKie_ELK/TOS_HWA/RightLane/TOS_HWA_RightLane/TOS_HWA_RightLane/TOS_HWA/HWA_RightLane ==
  Object_VX : Inport
  Object_VY : Inport  Port=2
  object_MovingState : Inport  Port=3
  PP_ObjMovingDirSignalProcessing : Inport  Port=4
  Object_HeadingAngle : Inport  Port=5
  Object_Type : Inport  Port=6
  TOS_TLJ_RightLaneConfirm_Flag : Inport  Port=7
  Object_DX : Inport  Port=8
  Object_DY : Inport  Port=9
  Object_Fus_Type : Inport  Port=10
  PP_ObjFusType_FC_FR_Confirm : Inport  Port=11
  PP_ObjFusType_FR_Confirm : Inport  Port=12
  PP_ObjFusType_FC_Confirm : Inport  Port=13
  VIE_EgoVelocity : Inport  Port=14
  Bus Creator : BusCreator  Inputs=14
  Bus Creator1 : BusCreator  Inputs=3
  Bus Creator2 : BusCreator  Inputs=10
  Bus Creator3 : BusCreator  Inputs=10
  Bus Creator4 : BusCreator  Inputs=10
  Bus Selector : BusSelector  OutputSignals=object_MovingState,PP_ObjMovingDirSignalProcessing,Object_HeadingAngle,Object_VX,Object_VY,VIE_EgoVelocity
  Bus Selector1 : BusSelector  OutputSignals=Object_VX,Object_VY,VIE_EgoVelocity
  Bus Selector2 : BusSelector  OutputSignals=HWA_MovState_InternalSig,HWA_InternalSig.Object_Fus_Type,HWA_InternalSig.TOS_TLJ_RightLaneConfirm_Flag,HWA_MovingDir_InternalSig,HWA_InternalSig.Object_DY,HWA_InternalSig.Object_DX
  Bus Selector3 : BusSelector  OutputSignals=HWA_InternalSig.object_MovingState,HWA_InternalSig.PP_ObjFusType_FR_Confirm,HWA_InternalSig.PP_ObjFusType_FC_Confirm,HWA_MovState_InternalSig,HWA_InternalSig.TOS_TLJ_RightLaneConfirm_Flag,HWA_MovingDir_InternalSig,HWA_InternalSig.Object_DX
  Bus Selector4 : BusSelector  OutputSignals=HWA_InternalSig.Object_DX
  Bus Selector5 : BusSelector  OutputSignals=HWA_InternalSig.Object_DX
  Bus Selector6 : BusSelector  OutputSignals=TOS_HWA_RightFront_TargConfirm_b,TOS_HWA_RightRear_TargConfirm_b,TOS_HWA_RightFront_FusType_ObserVale,TOS_HWA_InRightLane_Front_Flag_ObserVale,TOS_HWA_RightFront_TargMovDir_ObserVale,TOS_HWA_RightRear_MovState_ObserVale,TOS_HWA_RightRear_FusionType_ObserVale,TOS_HWA_InRightLane_Rear_Flag_ObserVale,TOS_HWA_RightRear_TargetMovingDir_ObserVale,TOS_HWA_RightRear_DyConfirm_ObserVale
  Compare To Constant1 : simulink/Logic and Bit Operations/Compare To Constant  relop=<=  const=P_TOS_EgoFrontDxThre_Val  OutDataTypeStr=boolean
      settings: AttributesFormatString=P_TOS_EgoFrontDxThre_Val = 120
  Compare To Constant14 : simulink/Logic and Bit Operations/Compare To Constant  relop=<  const=P_TOS_RefPoint_dx_m  OutDataTypeStr=boolean
      settings: AttributesFormatString=P_TOS_RefPoint_dx_m = 0
  Compare To Constant2 : simulink/Logic and Bit Operations/Compare To Constant  relop=>=  const=P_TOS_RefPoint_dx_m  OutDataTypeStr=boolean
      settings: AttributesFormatString=P_TOS_RefPoint_dx_m = 0
  Compare To Constant3 : simulink/Logic and Bit Operations/Compare To Constant  relop=>=  const=P_TOS_EgoRearDxThre_Val  OutDataTypeStr=boolean
      settings: AttributesFormatString=P_TOS_EgoRearDxThre_Val = -80
  HWA_MovState : Subsystem
  HWA_MovingDir : Subsystem
  HWA_RightLane_Default : Subsystem
  HWA_RightLane_Front : Subsystem
  HWA_RightLane_Rear : Subsystem
  Logical Operator1 : Logic  AllPortsSameDT=off  OutDataTypeStr=boolean
  Logical Operator2 : Logic  AllPortsSameDT=off  OutDataTypeStr=boolean
  Logical Operator3 : Logic  Operator=OR  AllPortsSameDT=off  OutDataTypeStr=boolean
  Switch : Switch  Criteria=u2 > Threshold
  Switch1 : Switch  Criteria=u2 > Threshold
  TOS_HWA_TargetInRightLane_b : Outport
  TOS_HWA_RightFront_TargConfirm_b : Outport  Port=2
  TOS_HWA_RightRear_TargConfirm_b : Outport  Port=3
  TOS_HWA_RightFront_FusType_ObserVale : Outport  Port=4
  TOS_HWA_InRightLane_Front_Flag_ObserVale : Outport  Port=5
  TOS_HWA_RightFront_TargMovDir_ObserVale : Outport  Port=6
  TOS_HWA_RightRear_MovState_ObserVale : Outport  Port=7
  TOS_HWA_RightRear_FusionType_ObserVale : Outport  Port=8
  TOS_HWA_InRightLane_Rear_Flag_ObserVale : Outport  Port=9
  TOS_HWA_RightRear_TargetMovingDir_ObserVale : Outport  Port=10
  TOS_HWA_RightRear_DyConfirm_ObserVale : Outport  Port=11
  wires:
  PP_ObjFusType_FC_Confirm/1 -> Bus Creator/13  "PP_ObjFusType_FC_Confirm"
  Bus Selector5/1 -> Compare To Constant1/1, Compare To Constant2/1  "<Object_DX>"
  Compare To Constant3/1 -> Logical Operator1/1
  Compare To Constant14/1 -> Logical Operator1/2
  Compare To Constant2/1 -> Logical Operator2/1
  Compare To Constant1/1 -> Logical Operator2/2
  Logical Operator1/1 -> Switch1/2
  Logical Operator2/1 -> Switch/2
  Object_VX/1 -> Bus Creator/1  "Object_VX"
  VIE_EgoVelocity/1 -> Bus Creator/14  "VIE_EgoVelocity"
  Object_VY/1 -> Bus Creator/2  "Object_VY"
  object_MovingState/1 -> Bus Creator/3  "object_MovingState"
  PP_ObjMovingDirSignalProcessing/1 -> Bus Creator/4  "PP_ObjMovingDirSignalProcessing"
  Object_HeadingAngle/1 -> Bus Creator/5  "Object_HeadingAngle"
  Object_Type/1 -> Bus Creator/6  "Object_Type"
  TOS_TLJ_RightLaneConfirm_Flag/1 -> Bus Creator/7  "TOS_TLJ_RightLaneConfirm_Flag"
  Object_DX/1 -> Bus Creator/8  "Object_DX"
  Object_Fus_Type/1 -> Bus Creator/10  "Object_Fus_Type"
  PP_ObjFusType_FC_FR_Confirm/1 -> Bus Creator/11  "PP_ObjFusType_FC_FR_Confirm"
  PP_ObjFusType_FR_Confirm/1 -> Bus Creator/12  "PP_ObjFusType_FR_Confirm"
  Bus Creator/1 -> Bus Selector1/1, Bus Selector/1, Bus Creator1/1  "HWA_InternalSig"
  Bus Selector/1 -> HWA_MovingDir/1(object_MovingState)  "<object_MovingState>"
  Bus Selector/2 -> HWA_MovingDir/2(PP_ObjMovingDirSignalProcessing)  "<PP_ObjMovingDirSignalProcessing>"
  Bus Selector/3 -> HWA_MovingDir/3(Object_HeadingAngle)  "<Object_HeadingAngle>"
  Bus Selector/4 -> HWA_MovingDir/4(Object_VX)  "<Object_VX>"
  Bus Selector/5 -> HWA_MovingDir/5(Object_VY)  "<Object_VY>"
  Bus Selector/6 -> HWA_MovingDir/6(VIE_EgoVelocity)  "<VIE_EgoVelocity>"
  Bus Selector1/1 -> HWA_MovState/1(Object_VX)  "<Object_VX>"
  Bus Selector1/2 -> HWA_MovState/2(Object_VY)  "<Object_VY>"
  Bus Selector1/3 -> HWA_MovState/3(VIE_EgoVelocity)  "<VIE_EgoVelocity>"
  HWA_MovState/1(HWA_MovState_InternalSig) -> Bus Creator1/3  "HWA_MovState_InternalSig"
  HWA_MovingDir/1(HWA_MovingDir_InternalSig) -> Bus Creator1/2  "HWA_MovingDir_InternalSig"
  Bus Creator1/1 -> Bus Selector4/1, Bus Selector2/1, Bus Selector5/1, Bus Selector3/1
  Object_DY/1 -> Bus Creator/9  "Object_DY"
  Bus Selector2/5 -> HWA_RightLane_Rear/5(Object_DY)  "<Object_DY>"
  Bus Selector2/4 -> HWA_RightLane_Rear/4(HWA_MovingDir_InternalSig)  "<HWA_MovingDir_InternalSig>"
  Bus Selector2/3 -> HWA_RightLane_Rear/3(TOS_TLJ_RightLaneConfirm_Flag)  "<TOS_TLJ_RightLaneConfirm_Flag>"
  Bus Selector2/2 -> HWA_RightLane_Rear/2(Object_Fus_Type)  "<Object_Fus_Type>"
  Bus Selector2/1 -> HWA_RightLane_Rear/1(HWA_MovState_InternalSig)  "<HWA_MovState_InternalSig>"
  Bus Selector3/1 -> HWA_RightLane_Front/1(object_MovingState)  "<object_MovingState>"
  Bus Selector3/2 -> HWA_RightLane_Front/2(PP_ObjFusType_FR_Confirm)  "<PP_ObjFusType_FR_Confirm>"
  Bus Selector3/3 -> HWA_RightLane_Front/3(PP_ObjFusType_FC_Confirm)  "<PP_ObjFusType_FC_Confirm>"
  Bus Selector3/4 -> HWA_RightLane_Front/4(HWA_MovState_InternalSig)  "<HWA_MovState_InternalSig>"
  Bus Selector3/5 -> HWA_RightLane_Front/5(TOS_TLJ_RightLaneConfirm_Flag)  "<TOS_TLJ_RightLaneConfirm_Flag>"
  Bus Selector3/6 -> HWA_RightLane_Front/6(HWA_MovingDir_InternalSig)  "<HWA_MovingDir_InternalSig>"
  Bus Selector2/6 -> HWA_RightLane_Rear/6(Object_DX)  "<Object_DX>"
  Bus Selector4/1 -> Compare To Constant14/1, Compare To Constant3/1  "<Object_DX>"
  HWA_RightLane_Front/1(TOS_HWA_RightFront_TargConfirm_b) -> Bus Creator2/1
  HWA_RightLane_Front/2(TOS_HWA_RightFront_FusType_ObserVale) -> Bus Creator2/2
  HWA_RightLane_Front/3(TOS_HWA_InRightLane_Front_Flag_ObserVale) -> Bus Creator2/3
  HWA_RightLane_Front/4(TOS_HWA_RightFront_TargMovDir_ObserVale) -> Bus Creator2/4
  HWA_RightLane_Front/5(TOS_HWA_RightRear_TargConfirm_b) -> Bus Creator2/5
  HWA_RightLane_Front/6(TOS_HWA_RightRear_MovState_ObserVale) -> Bus Creator2/6
  HWA_RightLane_Front/7(TOS_HWA_RightRear_FusionType_ObserVale) -> Bus Creator2/7
  HWA_RightLane_Front/8(TOS_HWA_InRightLane_Rear_Flag_ObserVale) -> Bus Creator2/8
  HWA_RightLane_Front/9(TOS_HWA_RightRear_TargetMovingDir_ObserVale) -> Bus Creator2/9
  HWA_RightLane_Front/10(TOS_HWA_RightRear_DyConfirm_ObserVale) -> Bus Creator2/10
  Bus Creator2/1 -> Switch/1
  HWA_RightLane_Rear/1(TOS_HWA_RightFront_TargConfirm_b) -> Bus Creator3/1
  HWA_RightLane_Rear/2(TOS_HWA_RightFront_FusType_ObserVale) -> Bus Creator3/2
  HWA_RightLane_Rear/3(TOS_HWA_InRightLane_Front_Flag_ObserVale) -> Bus Creator3/3
  HWA_RightLane_Rear/4(TOS_HWA_RightFront_TargMovDir_ObserVale) -> Bus Creator3/4
  HWA_RightLane_Rear/5(TOS_HWA_RightRear_TargConfirm_b) -> Bus Creator3/5
  HWA_RightLane_Rear/6(TOS_HWA_RightRear_MovState_ObserVale) -> Bus Creator3/6
  HWA_RightLane_Rear/7(TOS_HWA_RightRear_FusionType_ObserVale) -> Bus Creator3/7
  HWA_RightLane_Rear/8(TOS_HWA_InRightLane_Rear_Flag_ObserVale) -> Bus Creator3/8
  HWA_RightLane_Rear/9(TOS_HWA_RightRear_TargetMovingDir_ObserVale) -> Bus Creator3/9
  HWA_RightLane_Rear/10(TOS_HWA_RightRear_DyConfirm_ObserVale) -> Bus Creator3/10
  Bus Creator3/1 -> Switch1/1
  Switch1/1 -> Switch/3
  HWA_RightLane_Default/1(TOS_HWA_RightFront_TargConfirm_b) -> Bus Creator4/1
  HWA_RightLane_Default/2(TOS_HWA_RightFront_FusType_ObserVale) -> Bus Creator4/2
  HWA_RightLane_Default/3(TOS_HWA_InRightLane_Front_Flag_ObserVale) -> Bus Creator4/3
  HWA_RightLane_Default/4(TOS_HWA_RightFront_TargMovDir_ObserVale) -> Bus Creator4/4
  HWA_RightLane_Default/5(TOS_HWA_RightRear_TargConfirm_b) -> Bus Creator4/5
  HWA_RightLane_Default/6(TOS_HWA_RightRear_MovState_ObserVale) -> Bus Creator4/6
  HWA_RightLane_Default/7(TOS_HWA_RightRear_FusionType_ObserVale) -> Bus Creator4/7
  HWA_RightLane_Default/8(TOS_HWA_InRightLane_Rear_Flag_ObserVale) -> Bus Creator4/8
  HWA_RightLane_Default/9(TOS_HWA_RightRear_TargetMovingDir_ObserVale) -> Bus Creator4/9
  HWA_RightLane_Default/10(TOS_HWA_RightRear_DyConfirm_ObserVale) -> Bus Creator4/10
  Bus Creator4/1 -> Switch1/3
  Switch/1 -> Bus Selector6/1
  Bus Selector6/1 -> Logical Operator3/1, TOS_HWA_RightFront_TargConfirm_b/1  "<TOS_HWA_RightFront_TargConfirm_b>"
  Bus Selector6/2 -> Logical Operator3/2, TOS_HWA_RightRear_TargConfirm_b/1  "<TOS_HWA_RightRear_TargConfirm_b>"
  Bus Selector6/3 -> TOS_HWA_RightFront_FusType_ObserVale/1  "<TOS_HWA_RightFront_FusType_ObserVale>"
  Bus Selector6/4 -> TOS_HWA_InRightLane_Front_Flag_ObserVale/1  "<TOS_HWA_InRightLane_Front_Flag_ObserVale>"
  Bus Selector6/5 -> TOS_HWA_RightFront_TargMovDir_ObserVale/1  "<TOS_HWA_RightFront_TargMovDir_ObserVale>"
  Bus Selector6/6 -> TOS_HWA_RightRear_MovState_ObserVale/1  "<TOS_HWA_RightRear_MovState_ObserVale>"
  Bus Selector6/7 -> TOS_HWA_RightRear_FusionType_ObserVale/1  "<TOS_HWA_RightRear_FusionType_ObserVale>"
  Bus Selector6/8 -> TOS_HWA_InRightLane_Rear_Flag_ObserVale/1  "<TOS_HWA_InRightLane_Rear_Flag_ObserVale>"
  Bus Selector6/9 -> TOS_HWA_RightRear_TargetMovingDir_ObserVale/1  "<TOS_HWA_RightRear_TargetMovingDir_ObserVale>"
  Bus Selector6/10 -> TOS_HWA_RightRear_DyConfirm_ObserVale/1  "<TOS_HWA_RightRear_DyConfirm_ObserVale>"
  Logical Operator3/1 -> TOS_HWA_TargetInRightLane_b/1
  Bus Selector3/7 -> HWA_RightLane_Front/7(Object_DX)  "<Object_DX>"

== system PubIfDecisionTOS_MDL/TOS_20201112/TOS_2012080320/PIL_1029/ObjCutInOut_Prob/ObjectCutOut/CutOutProb_Calculate/CutOutProb_Calculate/CutOutProb_ScopeConstraint/ObjectCutoutMind/CutOutObjWidthConstraint/ObjectWidth_Check ==
  ObjectType : Inport
  Object_Width : Inport  Port=2
  Compare To Constant : simulink/Logic and Bit Operations/Compare To Constant  relop===  const=OFM_OBJ_TYPE_E.CAR  OutDataTypeStr=boolean
      settings: AttributesFormatString=OFM_OBJ_TYPE_E.CAR = 2
  Compare To Constant1 : simulink/Logic and Bit Operations/Compare To Constant  relop===  const=OFM_OBJ_TYPE_E.TRUCK  OutDataTypeStr=boolean
      settings: AttributesFormatString=OFM_OBJ_TYPE_E.TRUCK = 3
  Compare To Constant2 : simulink/Logic and Bit Operations/Compare To Constant  relop===  const=OFM_OBJ_TYPE_E.MOTORBIKE  OutDataTypeStr=boolean
      settings: AttributesFormatString=OFM_OBJ_TYPE_E.MOTORBIKE = 4
  Constant : Constant  Value=C_TOS_MotorbikeDefaultWidth_m  OutDataTypeStr=single
      settings: AttributesFormatString=C_TOS_MotorbikeDefaultWidth_m = 1
  Constant1 : Constant  Value=C_TOS_ObjectDefaultWidth_m  OutDataTypeStr=single
      settings: AttributesFormatString=C_TOS_ObjectDefaultWidth_m = 0.5
  Data Type Conversion : DataTypeConversion  OutDataTypeStr=Enum: OFM_OBJ_TYPE_E
  Logical Operator16 : Logic  Operator=OR  AllPortsSameDT=off  OutDataTypeStr=boolean
  Saturation : Saturate  UpperLimit=2.4  LowerLimit=1.6  OutDataTypeStr=single
  Switch : Switch  Criteria=u2 > Threshold
  Switch1 : Switch  Criteria=u2 > Threshold
  ObjectWidth : Outport
  wires:
  Constant1/1 -> Switch1/3
  Constant/1 -> Switch1/1
  Compare To Constant2/1 -> Switch1/2
  Switch1/1 -> Switch/3
  Saturation/1 -> Switch/1
  Switch/1 -> ObjectWidth/1
  Object_Width/1 -> Saturation/1
  ObjectType/1 -> Data Type Conversion/1
  Logical Operator16/1 -> Switch/2
  Compare To Constant1/1 -> Logical Operator16/2
  Data Type Conversion/1 -> Compare To Constant1/1, Compare To Constant2/1, Compare To Constant/1
  Compare To Constant/1 -> Logical Operator16/1

== system PubIfDecisionTOS_MDL/TOS_20201112/TOS_2012080320/PP1128/AAT-AdditionalAttributes/RoadEdge/RE_2020_12_07/RoadEdge_V2/RoadEdgeElementFinalJudge/EgoLeft_RoadEdgeElementsFinalJudge/Dy_Filter/If Action Subsystem ==
  Object_Dy : Inport
  Action Port : ActionPort  ActionPortLabel=if(u1|u2)
  Object_DyFilter : Outport
  wires:
  Object_Dy/1 -> Object_DyFilter/1

== system PubIfDecisionTOS_MDL/TOS_20201112/TOS_2012080320/PP1128/AAT-AdditionalAttributes/RoadEdge/RE_2020_12_07/RoadEdge_V2/RoadEdgeElementFinalJudge/EgoLeft_RoadEdgeElementsFinalJudge/Dy_Filter/Subsystem ==
  Object_Dy : Inport
  Object_Dy_K1 : Inport  Port=2
  Action Port : ActionPort  ActionPortLabel=else
  Abs : Abs
  Add : Sum  Inputs=+-
  Add1 : Sum
  Constant : Constant  Value=0.2  OutDataTypeStr=single
  Gain : Gain  Gain=0.5
  Relational Operator : RelationalOperator  Operator=<  OutDataTypeStr=boolean  RndMeth=Simplest
  Switch : Switch  Criteria=u2 ~= 0
  Object_DyFilter : Outport
  wires:
  Constant/1 -> Relational Operator/2
  Object_Dy/1 -> Switch/1, Add/1
  Gain/1 -> Add1/1
  Object_Dy_K1/1 -> Add1/2, Add/2
  Abs/1 -> Relational Operator/1
  Add/1 -> Gain/1, Abs/1
  Relational Operator/1 -> Switch/2
  Add1/1 -> Switch/3
  Switch/1 -> Object_DyFilter/1
